simulink model "filterbankFIRcompression"  (R2018a)
settings: Solver=FixedStepDiscrete  StartTime=0.0  StopTime=0.001  RelTol=1e-3
values from neighbouring files (symbols this model uses):
  fs = 35000    [filterbankProto.m]    (also in main.m = 44100; q2_computation.m = 20000)
  gainConsts = 10.^(requiredGainDB/10)    [main.m]
undefined symbols (not defined in the file or in its folder): fdesignblkfcn, gcbh
libraries: dspsrcs4 x1, dspxfrm3 x1, dspobslib x1
(part 3 of 3)

== system filterbankFIRcompression/Filter Bank OctaveFilterBlock/4th Octave/Bandpass Filter1 ==
  In : Inport
  Generated Filter Block : DiscreteFir  Tag=BlockMethodSubSystem  Coefficients=[0.000710536329578594235 0.000480231368416294668 0.000540923536368230007 0.000524201576661302224 0.00041851431816842925 0.000231560901313191141 -8.35020160617078832e-06 -0.000254900124502930551 -0.000453094722168828883 -0.000552258274331759807 -0.000521453451729783309 -0.000362971630165078558 -0.000121184341494637985 0.000117784174182406003 0.000236188702439771683 0.000106391569379987689 -0.000378805968729371259 -0.00127221433801458922 -0.00254269099733089822 -0.00405597379543916857 -0.00557232539498662017 -0.00676502416688979334 -0.0072635913509005055 -0.00671636518643186232 -0.00486103885830739112 -0.00159351103164123535 0.00296770840974742425 0.00846273648023987413 0.0142905850969617648 0.0196659298414647195 0.0237101728135856726 0.025574405800494044 0.0245786324611898983 0.020342303104531622 0.0128874318421906258 0.00269163130762194126 -0.00932199074144319552 -0.0218650010908490906 -0.0334261291642460115 -0.0424617623261350288 -0.0476085174179247117 -0.047887847868479147 -0.0428702341150930671 -0.0327721597674632548 -0.018467747201220238 -0.00140847204776089704 0.016542360783039816 0.0333389969370517375 0.0470144118585696658 0.0559390668035250199 0.0590393755506829557 0.0559390668035250199 0.0470144118585696658 0.0333389969370517375 0.016542360783039816 -0.00140847204776089704 -0.018467747201220238 -0.0327721597674632548 -0.0428702341150930671 -0.047887847868479147 -0.0476085174179247117 -0.0424617623261350288 -0.0334261291642460115 -0.0218650010908490906 -0.00932199074144319552 0.00269163130762194126 0.0128874318421906258 0.020342303104531622 0.0245786324611898983 0.025574405800494044 0.0237101728135856726 0.0196659298414647195 0.0142905850969617648 0.00846273648023987413 0.00296770840974742425 -0.00159351103164123535 -0.00486103885830739112 -0.00671636518643186232 -0.0072635913509005055 -0.00676502416688979334 -0.00557232539498662017 -0.00405597379543916857 -0.00254269099733089822 -0.00127221433801458922 -0.000378805968729371259 0.000106391569379987689 0.000236188702439771683 0.000117784174182406003 -0.000121184341494637985 -0.000362971630165078558 -0.000521453451729783309 -0.000552258274331759807 -0.000453094722168828883 -0.000254900124502930551 -8.35020160617078832e-06 0.000231560901313191141 0.00041851431816842925 0.000524201576661302224 0.000540923536368230007 0.000480231368416294668 0.000710536329578594235]  InputProcessing=Columns as channels (frame based)
  Out : Outport
  wires:
  In/1 -> Generated Filter Block/1
  Generated Filter Block/1 -> Out/1

== system filterbankFIRcompression/Filter Bank OctaveFilterBlock/4th Octave/Bandpass Filter2 ==
  In : Inport
  Generated Filter Block : DiscreteFir  Tag=BlockMethodSubSystem  Coefficients=[0.000660063968007304318 0.000362664224633989587 0.000413631548370213087 0.000430536325834472277 0.000405431575467652197 0.000335674548340531779 0.000224709284416333387 8.28061432437832422e-05 -7.39506217473550118e-05 -0.000224860365294900298 -0.000347996935854789761 -0.000422872953299833576 -0.000435264840810774126 -0.000380142447306632144 -0.00026540706276369561 -0.000112247838753902607 4.46670811529074712e-05 0.000160661250128451302 0.00018490286275318229 6.77886569879249009e-05 -0.000231277476419419813 -0.000734547883969277767 -0.00143841454837606597 -0.00230869166030908159 -0.00327727368234839765 -0.00424219720930289323 -0.00507361510846411536 -0.00562849123528509111 -0.00575677019582077239 -0.00532645863474424681 -0.00423782194333087534 -0.002441995563236923 4.2791099280662722e-05 0.00312322503769876109 0.00662626162874710781 0.0103060085160700272 0.0138558717698070068 0.0169324281160371064 0.019182779271531062 0.0202798100632131627 0.0199556074821101818 0.0180361408655775636 0.0144672258253103012 0.00933474324181769038 0.00287011131748247635 -0.00455489516060889055 -0.0124498997927794276 -0.0202379640112984351 -0.02730019705407127 -0.0330272255187208028 -0.0368730919939249252 -0.0384064787057949303 -0.0373559332063252633 -0.033642379468205072 -0.02739524596672566 -0.0189529261734629022 -0.0088427062489372845 0.00225645330798584327 0.0135640044396758367 0.0242611844710784591 0.0335561770280189062 0.0407514156070390154 0.0453006304965689263 0.0468569044160325882 0.0453006304965689263 0.0407514156070390154 0.0335561770280189062 0.0242611844710784591 0.0135640044396758367 0.00225645330798584327 -0.0088427062489372845 -0.0189529261734629022 -0.02739524596672566 -0.033642379468205072 -0.0373559332063252633 -0.0384064787057949303 -0.0368730919939249252 -0.0330272255187208028 -0.02730019705407127 -0.0202379640112984351 -0.0124498997927794276 -0.00455489516060889055 0.00287011131748247635 0.00933474324181769038 0.0144672258253103012 0.0180361408655775636 0.0199556074821101818 0.0202798100632131627 0.019182779271531062 0.0169324281160371064 0.0138558717698070068 0.0103060085160700272 0.00662626162874710781 0.00312322503769876109 4.2791099280662722e-05 -0.002441995563236923 -0.00423782194333087534 -0.00532645863474424681 -0.00575677019582077239 -0.00562849123528509111 -0.00507361510846411536 -0.00424219720930289323 -0.00327727368234839765 -0.00230869166030908159 -0.00143841454837606597 -0.000734547883969277767 -0.000231277476419419813 6.77886569879249009e-05 0.00018490286275318229 0.000160661250128451302 4.46670811529074712e-05 -0.000112247838753902607 -0.00026540706276369561 -0.000380142447306632144 -0.000435264840810774126 -0.000422872953299833576 -0.000347996935854789761 -0.000224860365294900298 -7.39506217473550118e-05 8.28061432437832422e-05 0.000224709284416333387 0.000335674548340531779 0.000405431575467652197 0.000430536325834472277 0.000413631548370213087 0.000362664224633989587 0.000660063968007304318]  InputProcessing=Columns as channels (frame based)
  Out : Outport
  wires:
  In/1 -> Generated Filter Block/1
  Generated Filter Block/1 -> Out/1

== system filterbankFIRcompression/Filter Bank OctaveFilterBlock/4th Octave/Bandpass Filter3 ==
  In : Inport
  Generated Filter Block : DiscreteFir  Tag=BlockMethodSubSystem  Coefficients=[0.000787331502509106213 0.000712646524578959312 0.00080733263120094656 0.000716818685482715871 0.000421733975543355823 -2.62032712578797442e-05 -0.000508755252751254446 -0.000871717056666874144 -0.000981365149126111084 -0.000786668501354213594 -0.000368661076257909709 5.08089081615513169e-05 0.000152109336404681906 -0.000380441370676968475 -0.00172796032965351299 -0.00380805836267096706 -0.00620294726378242678 -0.00817565816806206311 -0.00880470904152300983 -0.00722008769620908434 -0.00289396155425364647 0.00409650197993817727 0.0129033530108114535 0.0219340029530916969 0.0290867245209323298 0.0321742692167178782 0.0294680049938179679 0.0202173735581425498 0.00502276618867912583 -0.0140733482263830159 -0.0338310848896117497 -0.0503831341593400095 -0.0600230635359792833 -0.0600478088516138708 -0.0494521965606573854 -0.0292996680917166387 -0.00265467363998955243 0.0259359354665357547 0.0513146056273809936 0.0687604723729519918 0.0749708330126116207 0.0687604723729519918 0.0513146056273809936 0.0259359354665357547 -0.00265467363998955243 -0.0292996680917166387 -0.0494521965606573854 -0.0600478088516138708 -0.0600230635359792833 -0.0503831341593400095 -0.0338310848896117497 -0.0140733482263830159 0.00502276618867912583 0.0202173735581425498 0.0294680049938179679 0.0321742692167178782 0.0290867245209323298 0.0219340029530916969 0.0129033530108114535 0.00409650197993817727 -0.00289396155425364647 -0.00722008769620908434 -0.00880470904152300983 -0.00817565816806206311 -0.00620294726378242678 -0.00380805836267096706 -0.00172796032965351299 -0.000380441370676968475 0.000152109336404681906 5.08089081615513169e-05 -0.000368661076257909709 -0.000786668501354213594 -0.000981365149126111084 -0.000871717056666874144 -0.000508755252751254446 -2.62032712578797442e-05 0.000421733975543355823 0.000716818685482715871 0.00080733263120094656 0.000712646524578959312 0.000787331502509106213]  InputProcessing=Columns as channels (frame based)
  Out : Outport
  wires:
  In/1 -> Generated Filter Block/1
  Generated Filter Block/1 -> Out/1

== system filterbankFIRcompression/Filter Bank OctaveFilterBlock/5th Octave/Bandpass Filter1 ==
  In : Inport
  Generated Filter Block : DiscreteFir  Tag=BlockMethodSubSystem  Coefficients=[0.00104091797483246533 0.00117292590140649351 0.000889197178867677713 -5.47558220565934445e-05 -0.00105581072468561633 -0.00126993734640972193 -0.000460463792976197658 0.00036483088903188453 -0.000689227236600041255 -0.0048545614468881405 -0.0108429377827189734 -0.0142790649112275684 -0.00961648174968800055 0.00589001005015481714 0.0284539945020862994 0.047307034740027322 0.0491107476093929143 0.0257684310411888627 -0.0186907612150852449 -0.0670094081915204171 -0.0954760578341279226 -0.0859992831338889929 -0.037049322153253475 0.0332153066421266713 0.094386205223956271 0.118528095937172409 0.094386205223956271 0.0332153066421266713 -0.037049322153253475 -0.0859992831338889929 -0.0954760578341279226 -0.0670094081915204171 -0.0186907612150852449 0.0257684310411888627 0.0491107476093929143 0.047307034740027322 0.0284539945020862994 0.00589001005015481714 -0.00961648174968800055 -0.0142790649112275684 -0.0108429377827189734 -0.0048545614468881405 -0.000689227236600041255 0.00036483088903188453 -0.000460463792976197658 -0.00126993734640972193 -0.00105581072468561633 -5.47558220565934445e-05 0.000889197178867677713 0.00117292590140649351 0.00104091797483246533]  InputProcessing=Columns as channels (frame based)
  Out : Outport
  wires:
  In/1 -> Generated Filter Block/1
  Generated Filter Block/1 -> Out/1

== system filterbankFIRcompression/Filter Bank OctaveFilterBlock/5th Octave/Bandpass Filter2 ==
  In : Inport
  Generated Filter Block : DiscreteFir  Tag=BlockMethodSubSystem  Coefficients=[0.00135561766927554269 0.00183641062578695819 0.000895657920912027632 -0.00128416145068868085 -0.00248790199441557966 -0.00122421320096873345 0.000195133979586037236 -0.00307163487481588093 -0.0117559139584707019 -0.0170872868500709617 -0.0056427404214003489 0.025640733265371949 0.057950634843356684 0.0588079105062277938 0.00991002804479382444 -0.068005754341698782 -0.120597627195966339 -0.0993533621331094269 -0.00525970770089084338 0.103287289675446703 0.150873637626439683 0.103287289675446703 -0.00525970770089084338 -0.0993533621331094269 -0.120597627195966339 -0.068005754341698782 0.00991002804479382444 0.0588079105062277938 0.057950634843356684 0.025640733265371949 -0.0056427404214003489 -0.0170872868500709617 -0.0117559139584707019 -0.00307163487481588093 0.000195133979586037236 -0.00122421320096873345 -0.00248790199441557966 -0.00128416145068868085 0.000895657920912027632 0.00183641062578695819 0.00135561766927554269]  InputProcessing=Columns as channels (frame based)
  Out : Outport
  wires:
  In/1 -> Generated Filter Block/1
  Generated Filter Block/1 -> Out/1

== system filterbankFIRcompression/Filter Bank OctaveFilterBlock/5th Octave/Bandpass Filter3 ==
  In : Inport
  Generated Filter Block : DiscreteFir  Tag=BlockMethodSubSystem  Coefficients=[0.000884582308095480194 0.000870780307095067076 0.000848012585339726109 0.000462698932146210962 -0.000171370288053247658 -0.000762173546555128516 -0.000971002272625588877 -0.000645084665005441534 -6.26625629828922968e-06 0.000322456926781320406 -0.000441945506372254252 -0.00278782244015426083 -0.00641748539213879421 -0.00999905474017598675 -0.0113917109482768175 -0.00840857719289226507 9.01672573865113479e-05 0.0132084798673661238 0.0276463283734972344 0.0383073316765151911 0.0398770679933668215 0.0289216804599813741 0.00572864865713239996 -0.0249373784399444798 -0.0546816163773897607 -0.0738677306590229676 -0.0748465281281188444 -0.0548945716839916442 -0.0177156688303457925 0.0271963637366109436 0.0672739713077453727 0.0908193272405224683 0.0908193272405224683 0.0672739713077453727 0.0271963637366109436 -0.0177156688303457925 -0.0548945716839916442 -0.0748465281281188444 -0.0738677306590229676 -0.0546816163773897607 -0.0249373784399444798 0.00572864865713239996 0.0289216804599813741 0.0398770679933668215 0.0383073316765151911 0.0276463283734972344 0.0132084798673661238 9.01672573865113479e-05 -0.00840857719289226507 -0.0113917109482768175 -0.00999905474017598675 -0.00641748539213879421 -0.00278782244015426083 -0.000441945506372254252 0.000322456926781320406 -6.26625629828922968e-06 -0.000645084665005441534 -0.000971002272625588877 -0.000762173546555128516 -0.000171370288053247658 0.000462698932146210962 0.000848012585339726109 0.000870780307095067076 0.000884582308095480194]  InputProcessing=Columns as channels (frame based)
  Out : Outport
  wires:
  In/1 -> Generated Filter Block/1
  Generated Filter Block/1 -> Out/1

== system filterbankFIRcompression/Filter Bank OctaveFilterBlock/6th Octave/Bandpass Filter2 ==
  In : Inport
  Generated Filter Block : DiscreteFir  Tag=BlockMethodSubSystem  Coefficients=[0.00200608391046752307 0.00296182112284697078 -2.76446930316827056e-05 -0.00436306198413185988 -0.00343045138005433755 8.10391022939021302e-05 -0.00608795834538759014 -0.0189346990499320855 -0.00866814362833929174 0.0401795757156851105 0.0800848562720484908 0.0366037142511605532 -0.0830799022041095736 -0.157075771006374071 -0.0772702686389817872 0.100224558916550924 0.193113651985695661 0.100224558916550924 -0.0772702686389817872 -0.157075771006374071 -0.0830799022041095736 0.0366037142511605532 0.0800848562720484908 0.0401795757156851105 -0.00866814362833929174 -0.0189346990499320855 -0.00608795834538759014 8.10391022939021302e-05 -0.00343045138005433755 -0.00436306198413185988 -2.76446930316827056e-05 0.00296182112284697078 0.00200608391046752307]  InputProcessing=Columns as channels (frame based)
  Out : Outport
  wires:
  In/1 -> Generated Filter Block/1
  Generated Filter Block/1 -> Out/1
